simulink model "signalspecification_test"  (Simulink 8.4)
settings: Solver=VariableStepDiscrete  StartTime=0.0  StopTime=0  MaxStep=1  RelTol=1e-3
settings Model: Creator=arnaud  LastModifiedBy=arnaud
settings DataIOCC: ExternalInput=xin  SaveFormat=Structure

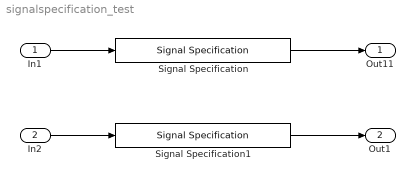
== system signalspecification_test ==
  In1 : Inport  OutDataTypeStr=Bus: BusA  PortDimensions=3  BusOutputAsStruct=on
  In2 : Inport  Port=2  OutDataTypeStr=double  PortDimensions=3  BusOutputAsStruct=on
  Signal Specification : SignalSpecification  OutDataTypeStr=Bus: BusA  BusOutputAsStruct=on
  Signal Specification1 : SignalSpecification  OutDataTypeStr=double  BusOutputAsStruct=on
  Out11 : Outport
  Out1 : Outport  Port=2
  wires:
  In1/1 -> Signal Specification/1
  Signal Specification/1 -> Out11/1
  In2/1 -> Signal Specification1/1
  Signal Specification1/1 -> Out1/1
